simulink model "MCLV2_dsPIC33EP256MC506_externalOpAmp_DataLog_R2017a"  (Simulink 8.9)
settings: Solver=FixedStepDiscrete  StartTime=0.0  StopTime=inf  FixedStep=.00005  RelTol=1e-3  EnableMultiTasking=on
undefined symbols (not defined in the file): A4, A8, B5, B6, C10, C5, C6, D5, DiscIntNeverNeededParam, F0, F1, Max, ms, P20, P24, P53, P54, P97, Pin, PWMmax, Resol, us
libraries: MCHP_Blockset x19, simulink x16, simulink_need_slupdate x1
(part 2 of 2)

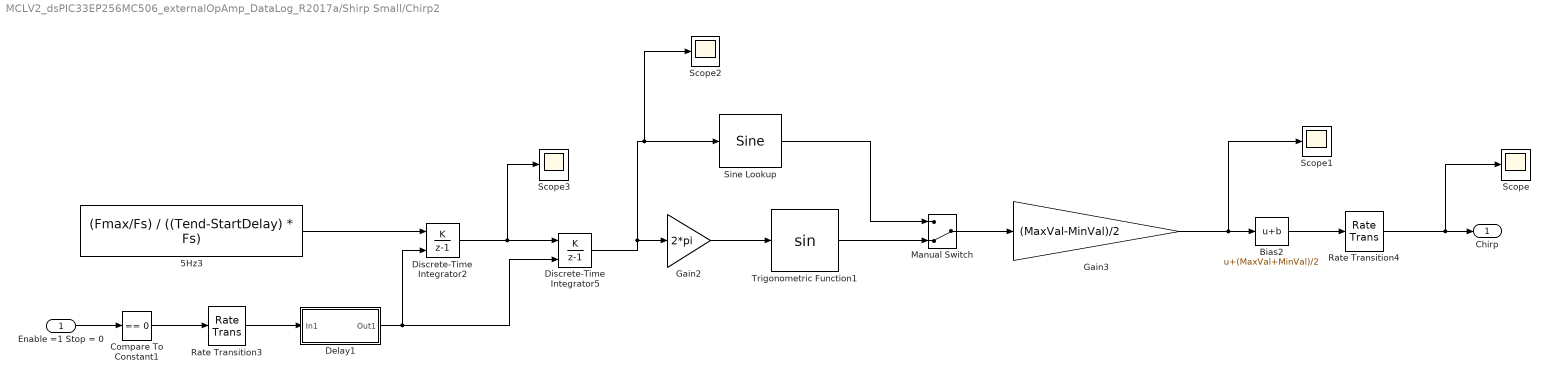
== system MCLV2_dsPIC33EP256MC506_externalOpAmp_DataLog_R2017a/Shirp Small/Chirp2 ==
  Enable =1 Stop = 0 : Inport
  5Hz3 : Constant  Value=(Fmax/Fs) / ((Tend-StartDelay) * Fs)  VectorParams1D=off  OutMin=0  OutMax=Fmax/Fs  OutDataTypeStr=fixdt(0,32)  SampleTime=1/Fs
  Bias2 : Bias  Bias=(MaxVal+MinVal)/2
  Compare To Constant1 : simulink/Logic and Bit Operations/Compare To Constant  relop===  const=0  OutDataTypeStr=boolean
  Delay1 : Subsystem
  Discrete-Time Integrator2 : DiscreteIntegrator  IntegratorMethod=Accumulation: Forward Euler  gainval=1  ExternalReset=level  InitialConditionSetting=State (most efficient)  SampleTime=1/Fs  OutMax=Fmax/Fs  OutDataTypeStr=fixdt(0,32)  ICPrevOutput=DiscIntNeverNeededParam  ICPrevScaledInput=DiscIntNeverNeededParam
      settings: LockScale=on
  Discrete-Time Integrator5 : DiscreteIntegrator  IntegratorMethod=Accumulation: Forward Euler  gainval=1  ExternalReset=level  InitialConditionSetting=State (most efficient)  SampleTime=1/Fs  OutDataTypeStr=fixdt(0,16,16)  ICPrevOutput=DiscIntNeverNeededParam  ICPrevScaledInput=DiscIntNeverNeededParam
      settings: LockScale=on
  Gain2 : Gain  Gain=2*pi  OutDataTypeStr=fixdt(0,16,13)
  Gain3 : Gain  Gain=(MaxVal-MinVal)/2  OutMin=[MinVal]  OutMax=[MaxVal]  OutDataTypeStr=fixdt(1,16)
  Manual Switch : ManualSwitch  CurrentSetting=0
  Rate Transition3 : RateTransition  Deterministic=off
  Rate Transition4 : RateTransition  Deterministic=off
  Scope{,1..3} (4 alike) : Scope
  Sine Lookup : simulink/Lookup Tables/Sine  Formula=sin(2*pi*u)  NumDataPoints=(2^10)+1  OutputWordLength=16  InternalRulePriority=Speed
      settings: SourceProductName=Simulink
  Trigonometric Function1 : Trigonometry  ApproximationMethod=CORDIC
  Chirp : Outport
  wires:
  Enable =1 Stop = 0/1 -> Compare To Constant1/1
  Discrete-Time Integrator2/1 -> Scope3/1, Discrete-Time Integrator5/1
  5Hz3/1 -> Discrete-Time Integrator2/1
  Discrete-Time Integrator5/1 -> Scope2/1, Sine Lookup/1, Gain2/1
  Compare To Constant1/1 -> Rate Transition3/1
  Rate Transition3/1 -> Delay1/1(In1)
  Delay1/1(Out1) -> Discrete-Time Integrator5/2, Discrete-Time Integrator2/2
  Gain2/1 -> Trigonometric Function1/1
  Gain3/1 -> Scope1/1, Bias2/1
  Bias2/1 -> Rate Transition4/1
  Rate Transition4/1 -> Scope/1, Chirp/1
  Trigonometric Function1/1 -> Manual Switch/2
  Manual Switch/1 -> Gain3/1
  Sine Lookup/1 -> Manual Switch/1

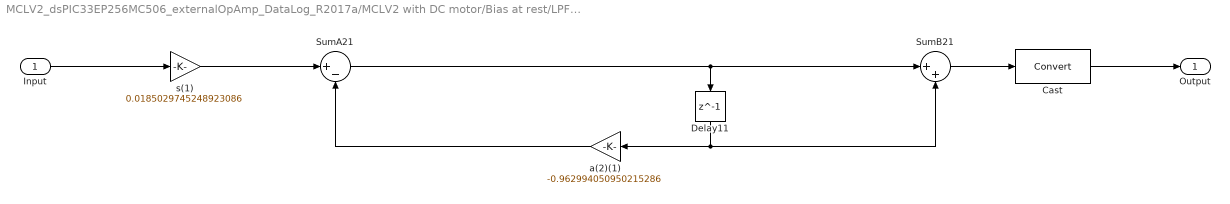
== system MCLV2_dsPIC33EP256MC506_externalOpAmp_DataLog_R2017a/MCLV2 with DC motor/Bias at rest/LPF_3Hz ==
  Input : Inport
  Cast : DataTypeConversion
  Delay11 : Delay  DelayLength=1  InitialCondition=0
  SumA21 : Sum  Inputs=|+-  RndMeth=Convergent  SaturateOnIntegerOverflow=on  OutDataTypeStr=Inherit: Same as first input
  SumB21 : Sum  Inputs=|++  RndMeth=Simplest  SaturateOnIntegerOverflow=on  OutDataTypeStr=Inherit: Same as first input
  a(2)(1) : Gain  Gain=-0.962994050950215286  ParamDataTypeStr=fixdt(1,16,14)  RndMeth=Simplest  OutDataTypeStr=Inherit: Same as input
  s(1) : Gain  Gain=0.0185029745248923086  ParamDataTypeStr=fixdt(1,16,20)  OutDataTypeStr=fixdt(1,16,16)  RndMeth=Convergent  SaturateOnIntegerOverflow=on
  Output : Outport
  wires:
  Cast/1 -> Output/1
  Input/1 -> s(1)/1
  SumB21/1 -> Cast/1
  Delay11/1 -> SumB21/2, a(2)(1)/1
  a(2)(1)/1 -> SumA21/2
  SumA21/1 -> Delay11/1, SumB21/1
  s(1)/1 -> SumA21/1

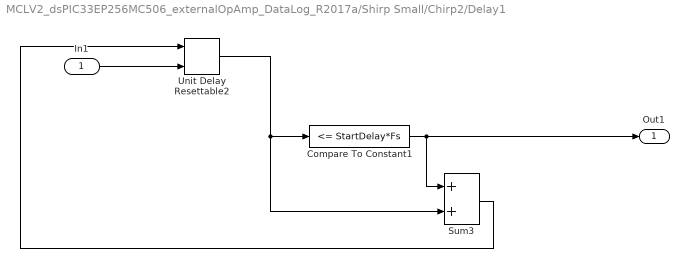
== system MCLV2_dsPIC33EP256MC506_externalOpAmp_DataLog_R2017a/Shirp Small/Chirp2/Delay1 ==
  In1 : Inport
  Compare To Constant1 : simulink/Logic and Bit Operations/Compare To Constant  relop=<=  const=StartDelay*Fs  OutDataTypeStr=boolean
  Sum3 : Sum  AccumDataTypeStr=uint16  OutDataTypeStr=Inherit: Same as accumulator
  Unit Delay Resettable2 : simulink_need_slupdate/Unit Delay Resettable  vinit=1  tsamp=inv(Fs)
      settings: SourceProductName=Simulink  SourceProductBaseCode=SL
  Out1 : Outport
  wires:
  Unit Delay Resettable2/1 -> Sum3/2, Compare To Constant1/1
  In1/1 -> Unit Delay Resettable2/2
  Sum3/1 -> Unit Delay Resettable2/1
  Compare To Constant1/1 -> Out1/1, Sum3/1
